simulink model "Solar_wind_hybrid_system_simulink"  (R2024a)
settings: Solver=VariableStepAuto  StartTime=0.0  StopTime=5  RelTol=1e-3
libraries: spsVoltageMeasurementLib x8, spsIGBTDiodeLib x7, spsSeriesRLCBranchLib x7, spsCurrentMeasurementLib x5, powerlib_extras x5, spsThreePhaseVIMeasurementLib x2, spsDiodeLib x2, spsPWMGeneratorDCDCLib x2, spsMosfetLib x1, spsPermanentMagnetSynchronousMachineLib x1, spsPVArrayLib x1, spsPWMGenerator2LevelLib x1
settings Model: Creator=shrin  LastModifiedBy=udhay
settings ModelReferenceCC: EnableRefExpFcnMdlSchedulingChecks=on
settings RTWCC: GPUComputeCapability=3.5

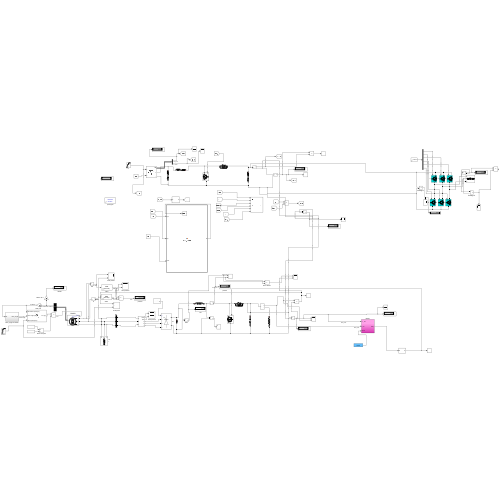
[thumbnail: Simulink's stored preview of the top-level diagram]
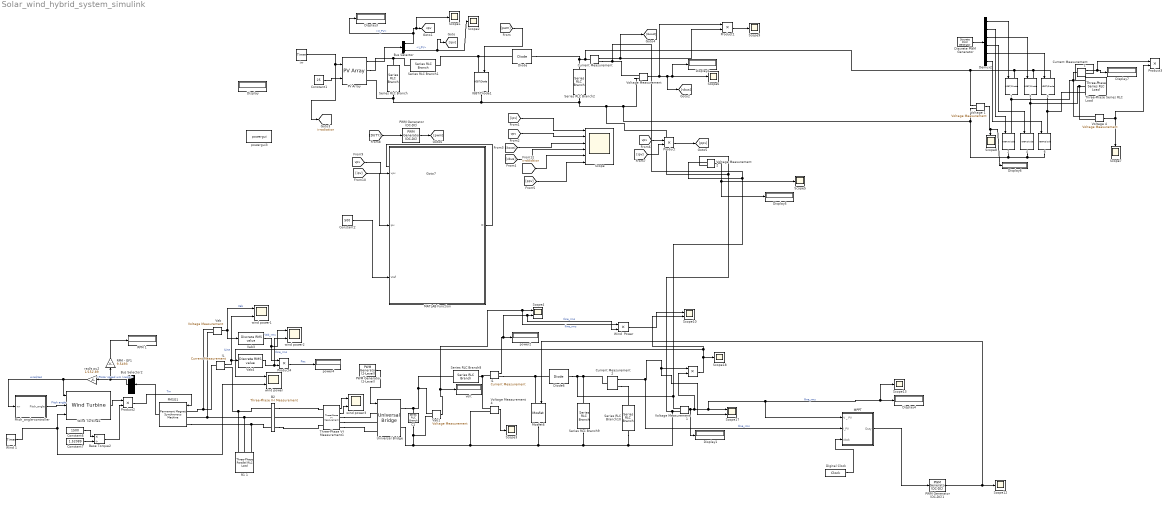
== system Solar_wind_hybrid_system_simulink ==
  " " : Product
  {1..6} (6 alike) : spsIGBTDiodeLib/IGBT//Diode  Ron=1e-3  Rs=1e5  Cs=inf  Measurements=off
  "B2 " : spsThreePhaseVIMeasurementLib/Three-Phase V-I Measurement  VoltageMeasurement=no  SetLabelV=on  LabelV=Vabc_B2  Vpu=off  VpuLL=off  CurrentMeasurement=no  SetLabelI=on  LabelI=Iabc_B2  Ipu=off  Pbase=100e6  Vbase=500e3  OutputType=Magnitude  PhasorSimulation=off  PSBequivalent=0
  Base Torque2 : Product  Inputs=*/  RndMeth=Zero
  Bus Selector : BusSelector  OutputSignals=V_PV,I_PV
  Bus Selector2 : BusSelector  OutputSignals=Rotor speed wm (rad/s)
  C1 : spsSeriesRLCBranchLib/Series RLC Branch  LConnTagsString=__new0  RConnTagsString=__new0  BranchType=C  Resistance=0.001  Inductance=1e-3  SetiL0=off  InitialCurrent=0  Capacitance=900e-6  Setx0=off  InitialVoltage=0  Measurements=None
  Constant1 : Constant  Value=25
  Constant2 : Constant  Value=500
  Constant6 : Constant  Value=1500
  Constant7 : Constant  Value=1.52089
  Current Measurement : spsCurrentMeasurementLib/Current Measurement  PhasorSimulation=off  OutputType=Complex  PSBequivalent=0
  Current Measurement1 : spsCurrentMeasurementLib/Current Measurement  PhasorSimulation=off  OutputType=Complex  PSBequivalent=0
  Current Measurement2 : spsCurrentMeasurementLib/Current Measurement  PhasorSimulation=off  OutputType=Complex  PSBequivalent=0
  Demux2 : Demux  Outputs=6
  Digital Clock : DigitalClock  SampleTime=0.001
  Diode : spsDiodeLib/Diode  Ron=0.001  Lon=0  Vf=0.8  IC=0  UseSnubber=0  Rs=500  Cs=250e-9  Measurements=off
  Diode6 : spsDiodeLib/Diode  Ron=0.001  Lon=0  Vf=0.8  IC=0  UseSnubber=0  Rs=500  Cs=250e-9  Measurements=off
  Discrete PWM Generator : powerlib_extras/Discrete  Control Blocks/Discrete PWM Generator  GeneratorMode="3-arm  bridge (6 pulses)"  Fc=1080  Ts=5e-6  Internal=on  mIndex=0.8  Freq=50  Phase=120
  Display{,1..7} (8 alike) : Display
  I1 : spsCurrentMeasurementLib/Current Measurement  PhasorSimulation=off  OutputType=Complex  PSBequivalent=0
  IGBT/Diode1 : spsIGBTDiodeLib/IGBT//Diode  Ron=1e-3  Rs=1e5  Cs=inf  Measurements=off
  IL : spsCurrentMeasurementLib/Current Measurement  PhasorSimulation=off  OutputType=Complex  PSBequivalent=0
  MATLAB Function : MATLAB Function  TreatAsAtomicUnit=on
  MPPT : Subsystem
  Mosfet6 : spsMosfetLib/Mosfet  Ron=0.1  Lon=0  Rd=0.01  Vfd=0.8  IC=0  Rs=1e5  Cs=inf  Measurements=off
  PMSG1 : spsPermanentMagnetSynchronousMachineLib/Permanent Magnet Synchronous Machine  NbPhases=3  FluxDistribution=Sinusoidal  RotorType=Round  MechanicalLoad=Torque Tm  PresetModel="16:  111 Nm 560 Vdc 3000 RPM - 126 Nm"  ShowDetailedParameters=on  MeasurementBus=off  Resistance=0.05  Inductance=8.5e-3  dqInductances=[0.0082 0.0082]  La=0.000635  MachineConstant=Flux linkage established by magnets (V.s)  Flux=0.192  VoltageCst=139.2998  TorqueCst=1.152  Flat=120  Mechanical=[0.011 0.001889 4 0]  PolePairs=4  InitialConditions=[0,0, 0,0]  InitialConditions5ph=[0 0 0 0 0 0]  RefAngle=90 degrees behind phase A axis (modified Park)  IterativeDiscreteModel=Trapezoidal non iterative  TsBlock=-1  TsPowergui=0
  PV Array : spsPVArrayLib/PV Array  Npar=7  Nser=3  PlotType=array @ 1000 W/m2 & specified temperatures  S_vec="[ 1000  500  100 ]"  Temp_C_vec="[ 45 25  ]"  ModuleName=Kyocera Solar KD130GX-LP  PlotWhenSelected=off  Pm=130.095  Ncell=36  Voc=22.1  Isc=8.06  Vm=17.7  Im=7.35  beta_Voc_pc=-0.32  alpha_Isc_pc=0.01  beta_Voc=-0.07072  alpha_Isc=0.000806  IL=8.1611  I0=5.7398e-11  nI=0.93281  Rsh=42.8077  Rs=0.24594  RobustModel=off  RobustCellTemperature=313.3991  BAL=on  Tc=1e-6  Tfilter=5e-5
  PWM Generator (2-Level) : spsPWMGenerator2LevelLib/PWM Generator (2-Level)  ModulatorType=Three-phase bridge (6 pulses)  ModulatorMode=Unsynchronized  Fc=3000  Pc=90  nF=27  MinMax="[ -1  1 ]"  SamplingTechnique=Natural  ModulatingSignals=on  m=0.8  Freq=50  Phase=0  Ts=0  ShowCarrierOutport=off
  PWM Generator (DC-DC) : spsPWMGeneratorDCDCLib/PWM Generator (DC-DC)  Fsw=5000  Ts=10e-6
  PWM Generator (DC-DC)1 : spsPWMGeneratorDCDCLib/PWM Generator (DC-DC)  Fsw=5000  Ts=0
  Pitch_angle-controller : Subsystem
  Product : Product
  Product1 : Product
  Product2 : Product  RndMeth=Zero
  Product3 : Product
  Product4 : Product  RndMeth=Zero
  R1 1 : spsThreePhaseParallelRLCLoadLib/Three-Phase Parallel RLC Load  LConnTagsString=A|B|C  Configuration=Y (grounded)  NominalVoltage=220  Vabc=[1e3 1e3 1e3]  Vabcp=[1e3 1e3 1e3]  NominalFrequency=50  UnbalancedPower=off  ActivePower=5000  InductivePower=0  CapacitivePower=0  Pabc=[9e3 9e3 9e3]  QLabc=[100 90 110]  QCabc=[100 90 110]  Pabcp=[10e3 9e3 11e3]  QLabcp=[100 90 110]  QCabcp=[100 90 110]  Measurements=None  LoadType=constant Z
  RPM - GF1 : Gain  Gain=9.5493  SaturateOnIntegerOverflow=on  OutDataTypeStr=Inherit: Same as input  ParamDataTypeStr=Inherit: Same as input
  RPM 1 : Display
  Scope : Scope  NumInputPorts=6
  Scope{1..3,5..9,12..13,18} (11 alike) : Scope
  Scope10 : Scope  NumInputPorts=2
  Scope17 : Scope  NumInputPorts=2
  Scope4 : Scope  NumInputPorts=2
  Series RLC Branch : spsSeriesRLCBranchLib/Series RLC Branch  LConnTagsString=__new0  RConnTagsString=__new0  BranchType=RC  Resistance=1e-6  Inductance=1e-3  SetiL0=off  InitialCurrent=0  Capacitance=1000e-6  Setx0=off  InitialVoltage=0  Measurements=None
  Series RLC Branch1 : spsSeriesRLCBranchLib/Series RLC Branch  LConnTagsString=__new0  RConnTagsString=__new0  BranchType=RL  Resistance=0.1  Inductance=1e-3  SetiL0=off  InitialCurrent=0  Capacitance=1000e-6  Setx0=off  InitialVoltage=0  Measurements=None
  Series RLC Branch10 : spsSeriesRLCBranchLib/Series RLC Branch  LConnTagsString=__new0  RConnTagsString=__new0  BranchType=R  Resistance=6  Inductance=1e-3  SetiL0=off  InitialCurrent=0  Capacitance=1e-6  Setx0=off  InitialVoltage=0  Measurements=None
  Series RLC Branch2 : spsSeriesRLCBranchLib/Series RLC Branch  LConnTagsString=__new0  RConnTagsString=__new0  BranchType=RC  Resistance=1e-4  Inductance=1e-3  SetiL0=off  InitialCurrent=0  Capacitance=3300e-6  Setx0=off  InitialVoltage=0  Measurements=None
  Series RLC Branch8 : spsSeriesRLCBranchLib/Series RLC Branch  LConnTagsString=__new0  RConnTagsString=__new0  BranchType=L  Resistance=1  Inductance=0.4e-1  SetiL0=off  InitialCurrent=0  Capacitance=1e-6  Setx0=off  InitialVoltage=0  Measurements=None
  Series RLC Branch9 : spsSeriesRLCBranchLib/Series RLC Branch  LConnTagsString=__new0  RConnTagsString=__new0  BranchType=C  Resistance=110  Inductance=1e-3  SetiL0=off  InitialCurrent=0  Capacitance=750e-6  Setx0=off  InitialVoltage=0  Measurements=None
  Three-Phase Series RLC Load : spsThreePhaseSeriesRLCLoadLib/Three-Phase Series RLC Load  LConnTagsString=A|B|C  Configuration=Y (grounded)  NominalVoltage=1000  Vabc=[1e3 1e3 1e3]  Vabcp=[1e3 1e3 1e3]  NominalFrequency=60  UnbalancedPower=off  ActivePower=10e3  InductivePower=100  CapacitivePower=100  Pabc=[10e3 9e3 11e3]  QLabc=[100 90 110]  QCabc=[100 90 110]  Pabcp=[10e3 9e3 11e3]  QLabcp=[100 90 110]  QCabcp=[100 90 110]  Measurements=None  LoadType=constant Z
  Three-Phase V-I Measurement1 : spsThreePhaseVIMeasurementLib/Three-Phase V-I Measurement  VoltageMeasurement=phase-to-phase  SetLabelV=off  LabelV=Vabc  Vpu=off  VpuLL=off  CurrentMeasurement=yes  SetLabelI=off  LabelI=Iabc  Ipu=off  Pbase=100e6  Vbase=500e3  OutputType=Complex  PhasorSimulation=off  PSBequivalent=0
  Universal Bridge : spsUniversalBridgeLib/Universal Bridge  Arms=3  SnubberResistance=1e5  SnubberCapacitance=inf  Device=Thyristors  Ron=1e-3  Lon=0  ForwardVoltages="[  0  0  ]"  ForwardVoltage=0.8  GTOparameters=[ 10e-6 , 20e-6 ]  IGBTparameters=[ 1e-6 , 2e-6 ]  Measurements=None  Measurements_2=None  converterType=Rectifier
  Vab : spsVoltageMeasurementLib/Voltage Measurement  PhasorSimulation=off  OutputType=Complex  PSBequivalent=0
  Vab1 : spsVoltageMeasurementLib/Voltage Measurement  PhasorSimulation=off  OutputType=Complex  PSBequivalent=0
  Vab3 : powerlib_extras/Discrete Measurements/Discrete  RMS value  Freq=50  Mag_Init=0  Ts=20e-6
  Vab4 : powerlib_extras/Discrete Measurements/Discrete  RMS value  Freq=50  Mag_Init=0  Ts=20e-6
  Voltage 1 : spsVoltageMeasurementLib/Voltage Measurement  PhasorSimulation=off  OutputType=Complex  PSBequivalent=0
  Voltage 4 : spsVoltageMeasurementLib/Voltage Measurement  PhasorSimulation=off  OutputType=Complex  PSBequivalent=0
  Voltage Measurement{,1..2,4} (4 alike) : spsVoltageMeasurementLib/Voltage Measurement  PhasorSimulation=off  OutputType=Complex  PSBequivalent=0
  Wind  Power : Product
  Wind 1 : powerlib_extras/Control  Blocks/Timer  t="[0 0.5 1 2  4 ]"  e=[5 7 11 12 12]
  Wind Turbine1 : spsWindTurbineLib/Wind Turbine  Pnom=80000  Pelec_base=80000/0.9  wind_base=12  P_wind_base=0.73  speed_nom=1.2  pitch_angle=0  c1_c6="[0.51763          116          0.4            5           21     0.006795]"  cp_nom=0.48  lambda_nom=8.1
  irr : powerlib_extras/Control  Blocks/Timer  t="[0 0.5 1 2  4 ]"  e=[250 500 750 1000 1000]
  power2 : Display
      settings: SampleTime=1e-3
  power4 : Display
      settings: SampleTime=1e-3
  powergui3 : spspowerguiLib/powergui  Priority=1  SimulationMode=Discrete  SampleTime=5e-6  frequency=60  Iterations=50  frequencyindice=0  Pbase=100e6  ErrMax=1e-4  UnitsV=kV  UnitsW=MW  buscounter=0  FunctionMessages=off  echomessages=off  EnableUseOfTLC=off  CurrentSourceSwitches=off  DisableSnubberDevices=off  DisableRonSwitches=off  DisableVfSwitches=off  DisplayEquations=off  AutomaticDiscreteSolvers=off  SolverType=Tustin/Backward Euler (TBE)  Interpol=off  ExternalGateDelay=off  methode=off  Ts=100  x0status=blocks  SPID=on  SwTol=0  HookPort=off  NonlinearTolerance=1e-4  nMaxIteration=100  ContinueOnMaxIteration=off  RestoreLinks=warning  ResistiveCurrentMeasurement=off  Frange=[0:2:500]  Ylog=off  Xlog=on  ShowGrid=off  save=off  variable=ZData  structure=0  ZoomFFT=off  StartTime=0.0  cycles=1  DisplayStyle=1  fundamental=60  FreqAxis=off  MaxFrequency=1000  frequencyindicesteady=1  RmsSteady=1  display=off
  rad/s pu2 : Gain  Gain=1/152.89  SaturateOnIntegerOverflow=on  OutDataTypeStr=Inherit: Same as input  ParamDataTypeStr=Inherit: Same as input
  volt : Display
      settings: SampleTime=1e-3
  wind power{,1..3} (4 alike) : Scope  NumInputPorts=2
  tag scope: irradiation=global, vpv=global
  wires:
  irr/1 -> [irradiation], PV Array/1
  Constant1/1 -> PV Array/2
  PV Array/1 -> Bus Selector/1
  Bus Selector/1 -> Display3/1, Scope1/1, [vpv]  "<V_PV>"
  Current Measurement/1 -> Product1/2, [iboost]
  Bus Selector/2 -> Scope2/1, [ipv]  "<I_PV>"
  [pwm] -> IGBT/Diode1/1
  [ipv] -> Scope/1
  [vpv] -> Scope/2
  [iboost] -> Scope/3
  [vbus] -> Scope/4
  [ppv] -> Scope/6
  Product/1 -> [ppv]
  [vpv] -> Product/1
  [ipv] -> Product/2
  PWM Generator (DC-DC)/1 -> [pwm]
  [DUTY] -> PWM Generator (DC-DC)/1
  [vpv] -> MATLAB Function/1(vpv)
  [ipv] -> MATLAB Function/2(ipv)
  MATLAB Function/1(D) -> [DUTY]
  [irradiation] -> Scope/5
  Voltage Measurement/1 -> Product1/1, Display2/1, Scope6/1, [vbus]
  PWM Generator (DC-DC)1/1 -> Mosfet6/1, Scope12/1
  PMSG1/1 -> Bus Selector2/1
  Pitch_angle-controller/1(Pitch_angle) -> Wind Turbine1/2  "Pitch angle"
  Voltage Measurement4/1 -> Scope3/1
  Three-Phase V-I Measurement1/2 -> wind power3/2
  Vab1/1 -> volt/1, Wind  Power/1, Scope4/1  "Iline_rms"
  " "/1 -> wind power/1, Scope10/2, Scope18/1
  Vab4/1 -> wind power2/2, Product4/2  "Iline_rms"
  Product4/1 -> power4/1  "Pac"
  IL/1 -> Vab4/1, wind power1/2  "ILine"
  Wind 1/1 -> wind power/2, Wind Turbine1/3
  Wind Turbine1/1 -> Product2/1
  RPM - GF1/1 -> RPM 1/1
  Constant7/1 -> Base Torque2/2
  Vab/1 -> Vab3/1, wind power1/1  "Vab"
  Vab3/1 -> Product4/1, wind power2/1  "Vab_rms"
  Bus Selector2/1 -> RPM - GF1/1, rad/s pu2/1  "<Rotor speed wm (rad/s)>"
  I1/1 -> Wind  Power/2, Scope4/2, power2/1  "Iline_rms"
  Wind  Power/1 -> Scope10/1
  Constant6/1 -> Base Torque2/1
  Base Torque2/1 -> Product2/2
  rad/s pu2/1 -> Wind Turbine1/1, Pitch_angle-controller/1(wr)  "wrad/sec"
  Three-Phase V-I Measurement1/1 -> wind power3/1
  PWM Generator (2-Level)/1 -> Universal Bridge/1
  Product2/1 -> PMSG1/1  "Tm"
  Voltage Measurement2/1 -> Display5/1, Scope5/1
  Voltage 1/1 -> Scope8/1, Display6/1
  Demux2/5 -> 5/1
  Demux2/2 -> 2/1
  Demux2/4 -> 4/1
  Discrete PWM Generator/1 -> Demux2/1
  Demux2/6 -> 6/1
  Voltage 4/1 -> Scope7/1, Product3/2
  Demux2/3 -> 3/1
  Demux2/1 -> 1/1
  Product1/1 -> Scope9/1
  Current Measurement1/1 -> Product3/1, Display7/1
  Voltage Measurement1/1 -> Display1/1, " "/2, MPPT/1("V _ PV "), Scope13/1, Display4/1, Scope17/1  "Iline_rms"
  Current Measurement2/1 -> MPPT/2(I_PV), Scope17/2, " "/1  "Iline_rms"
  Digital Clock/1 -> MPPT/3(clock)
  MPPT/1(Duty) -> PWM Generator (DC-DC)1/1
  Constant2/1 -> MATLAB Function/3(Vref)
  connections:
  PV Array/RConn1 -- Series RLC Branch/LConn1 -- Series RLC Branch1/RConn1
  Series RLC Branch1/LConn1 -- IGBT/Diode1/LConn1 -- Diode/LConn1
  Voltage 1/LConn1 -- Diode/RConn1 -- Series RLC Branch2/LConn1 -- Current Measurement/LConn1 -- 5/LConn1 -- 3/LConn1 -- 1/LConn1
  I1/RConn1 -- Diode6/LConn1 -- Mosfet6/LConn1
  Series RLC Branch8/RConn1 -- Voltage Measurement4/LConn1 -- I1/LConn1
  "B2 "/LConn1 -- R1 1/LConn1 -- IL/RConn1
  Vab/LConn2 -- R1 1/LConn2 -- "B2 "/LConn2 -- PMSG1/LConn2
  C1/LConn1 -- Universal Bridge/RConn1 -- Series RLC Branch8/LConn1 -- Vab1/LConn1
  Vab/LConn1 -- IL/LConn1 -- PMSG1/LConn1
  PMSG1/LConn3 -- R1 1/LConn3 -- "B2 "/LConn3
  Three-Phase V-I Measurement1/LConn2 -- "B2 "/RConn2
  Three-Phase V-I Measurement1/RConn1 -- Universal Bridge/LConn1
  "B2 "/RConn3 -- Three-Phase V-I Measurement1/LConn3
  "B2 "/RConn1 -- Three-Phase V-I Measurement1/LConn1
  Three-Phase V-I Measurement1/RConn2 -- Universal Bridge/LConn2
  Three-Phase V-I Measurement1/RConn3 -- Universal Bridge/LConn3
  Current Measurement2/RConn1 -- Series RLC Branch10/LConn1
  Voltage Measurement2/LConn1 -- Current Measurement/RConn1 -- Voltage Measurement/LConn1 -- Voltage Measurement1/LConn1 -- Current Measurement2/LConn1 -- Series RLC Branch9/LConn1 -- Diode6/RConn1
  Voltage 1/LConn2 -- Series RLC Branch10/RConn1 -- Voltage Measurement4/LConn2 -- C1/RConn1 -- Vab1/LConn2 -- Universal Bridge/RConn2 -- Mosfet6/RConn1 -- Series RLC Branch9/RConn1 -- Voltage Measurement1/LConn2 -- Voltage Measurement2/LConn2 -- Series RLC Branch/RConn1 -- PV Array/RConn2 -- IGBT/Diode1/RConn1 -- Series RLC Branch2/RConn1 -- Voltage Measurement/LConn2 -- 6/RConn1 -- 4/RConn1 -- 2/RConn1
  3/RConn1 -- Voltage 4/LConn2 -- Three-Phase Series RLC Load/LConn2 -- 4/LConn1
  1/RConn1 -- Current Measurement1/LConn1 -- Voltage 4/LConn1 -- 2/LConn1
  5/RConn1 -- 6/LConn1 -- Three-Phase Series RLC Load/LConn3
  Three-Phase Series RLC Load/LConn1 -- Current Measurement1/RConn1

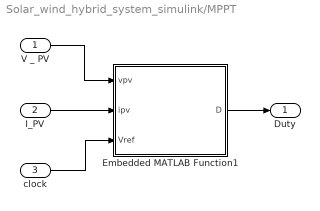
== system Solar_wind_hybrid_system_simulink/MPPT ==
  "V _ PV " : Inport
  I_PV : Inport  Port=2
  clock : Inport  Port=3
  Embedded MATLAB Function1 : MATLAB Function  TreatAsAtomicUnit=on
  Duty : Outport  VectorParamsAs1DForOutWhenUnconnected=off
  wires:
  I_PV/1 -> Embedded MATLAB Function1/2(ipv)
  "V _ PV "/1 -> Embedded MATLAB Function1/1(vpv)
  clock/1 -> Embedded MATLAB Function1/3(Vref)
  Embedded MATLAB Function1/1(D) -> Duty/1

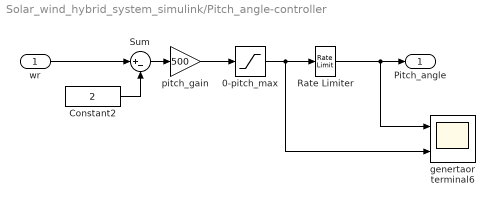
== system Solar_wind_hybrid_system_simulink/Pitch_angle-controller ==
  wr : Inport
  0-pitch_max : Saturate  UpperLimit=100  LowerLimit=0
  Constant2 : Constant  Value=2
  "Rate Limiter   " : RateLimiter  RisingSlewLimit=4  FallingSlewLimit=-4
  Sum : Sum  Inputs=|+-  SaturateOnIntegerOverflow=on
  genertaor terminal6 : Scope  NumInputPorts=2
  pitch_gain : Gain  Gain=500  SaturateOnIntegerOverflow=on  OutDataTypeStr=Inherit: Same as input  ParamDataTypeStr=Inherit: Same as input
  Pitch_angle : Outport  VectorParamsAs1DForOutWhenUnconnected=off
  wires:
  wr/1 -> Sum/1
  0-pitch_max/1 -> genertaor terminal6/2, "Rate Limiter   "/1
  Constant2/1 -> Sum/2
  Sum/1 -> pitch_gain/1
  pitch_gain/1 -> 0-pitch_max/1
  "Rate Limiter   "/1 -> genertaor terminal6/1, Pitch_angle/1

== matlab function Solar_wind_hybrid_system_simulink/MPPT/Embedded MATLAB Function1 ==
  settings: updateMethod=DISCRETE
  data: vpv input; ipv input; Vref input; D output
function D = mppt_honeybee_pid(vpv, ipv, Vref)
    persistent Dprev vprev pprev iprev bees power_bees pid_integral pid_prev_error
    
    % Parameters
    num_bees = 10;
    num_iterations = 100;
    deltaD = 125e-6;
    Kp = 0.1;  % Proportional gain
    Ki = 0.01; % Integral gain
    Kd = 0.01; % Derivative gain
    
    % Initialize persistent variables
    if isempty(Dprev)
        Dprev = 0.7;
        vprev = 190;
        pprev = 2000;
        iprev = 0;
        bees = rand(1, num_bees);  % Random initial duty cycles
        power_bees = zeros(1, num_bees);
        pid_integral = 0;
        pid_prev_error = 0;
    end
    
    Ppv = vpv * ipv;
    
    % Evaluate the power for each bee
    for i = 1:num_bees
        power_bees(i) = bees(i) * ipv * vpv; % Simplified power calculation
    end
    
    % Select the best bee
    [~, best_bee_index] = max(power_bees);
    D = bees(best_bee_index);
    
    % Perform neighborhood search around the best bee
    for iter = 1:num_iterations
        for i = 1:num_bees
            if i ~= best_bee_index
                bees(i) = bees(best_bee_index) + (rand - 0.5) * deltaD;
                bees(i) = max(0, min(bees(i), 1)); % Ensure D is within bounds [0, 1]
            end
        end
        
        % Evaluate the power for each bee
        for i = 1:num_bees
            power_bees(i) = bees(i) * ipv * vpv; % Simplified power calculation
        end
        
        % Select the best bee
        [~, best_bee_index] = max(power_bees);
        D = bees(best_bee_index);
    end
    
    % PID controller for fine-tuning
    error = Vref - vpv;
    pid_integral = pid_integral + error;
    pid_derivative = error - pid_prev_error;
    
    % PID output for duty cycle adjustment
    D = D + Kp * error + Ki * pid_integral + Kd * pid_derivative;
    D = max(0, min(D, 1)); % Ensure D is within bounds [0, 1]
    
    % Update previous values
    Dprev = D;
    vprev = vpv;
    pprev = Ppv;
    iprev = ipv;
    pid_prev_error = error;
end

== matlab function Solar_wind_hybrid_system_simulink/MATLAB Function ==
  data: vpv input; D output; ipv input; Vref input
function D = mppt_pando(vpv, ipv, Vref)
    persistent Dprev vprev pprev deltaD direction
    
    % Parameters
    deltaD = 125e-6; % Perturbation size
    if nargin < 3
        Vref = 200; % Default reference voltage if not provided
    end
    
    % Initialize persistent variables
    if isempty(Dprev)
        Dprev = 0.7; % Initial duty cycle
        vprev = 190; % Initial voltage
        pprev = 2000; % Initial power
        direction = 1; % Direction of perturbation: 1 for increase, -1 for decrease
    end
    
    % Compute current power
    Ppv = vpv * ipv;
    
    % Perturb and Observe algorithm
    if (Ppv - pprev) > 0
        % Power has increased
        if (vpv - vprev) > 0
            % Voltage has increased
            D = Dprev + deltaD * direction;
        else
            % Voltage has decreased
            D = Dprev - deltaD * direction;
        end
        % Change direction for the next perturbation
        direction = -direction;
    else
        % Power has decreased
        if (vpv - vprev) > 0
            % Voltage has increased
            D = Dprev - deltaD * direction;
        else
            % Voltage has decreased
            D = Dprev + deltaD * direction;
        end
    end
    
    % Ensure D is within bounds [0, 1]
    D = max(0, min(D, 1));
    
    % Update persistent variables
    Dprev = D;
    vprev = vpv;
    pprev = Ppv;
end
